simulink model "Corrado_simscape"  (R2023b)
settings: Solver=ode15s  StartTime=0.0  StopTime=15  RelTol=1e-2  AbsTol=1e-2  EnableMultiTasking=on
libraries: ee_lib x18, fl_lib x18, sm_lib x17, nesl_utility x7, simulink_extras x6
(part 2 of 2)

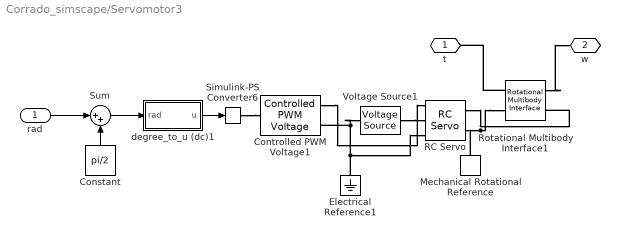
== system Corrado_simscape/Servomotor3 ==
  rad : Inport
  Constant : Constant  Value=pi/2
  Controlled PWM Voltage1 : ee_lib/Integrated Circuits/Controlled PWM Voltage  F=50 Hz  TD=0 s  pulse_width_offset=0 s  pulse_min=0 us  pwm_or_av=ee.enum.pwm_or_av.pwm  event_type=1  sample_time=5e-6 s  Vmin=0 V  Vmax=5 V  Vm=5 V  u_min=0  u_max=1
      settings: InternalSimscapePortConfiguration="{\"Bottom\":[],\"Left\":[{\"id\":\"u\",\"label\":\"u\",\"type\":\"input\"}],\"Right\":[{\"id\":\"p2\",\"label\":\"PWM\",\"type\":\"foundation.electrical.electrical\"},{\"id\":\"n2\",\"label\":\"REF\",\"type\":\"foundation.electrical.electrical\"}],\"Top\":[]}"
  Electrical Reference1 : fl_lib/Electrical/Electrical Elements/Electrical Reference
  Mechanical Rotational Reference : fl_lib/Mechanical/Rotational Elements/Mechanical Rotational Reference
  RC Servo : ee_lib/Electromechanical/Brushed Motors/RC Servo  stall_torque=15 cm*kg  time_60=0.13 s  nominal_voltage=6 V  rotational_range=[0, 180] deg  pulse_width_range=[600, 2400] us  threshold=3 V  R_s=18 kOhm  resolution=0.1 deg  angle_meas_error=0 deg  backdrive_torque=0.5 cm*kg  ratio=320  inertia=0.01 cm^2*g  endstop_angles=[-5, 185] deg  endstop_stiffness=1e6 N*m/rad  endstop_damping=0.01 N*m*s/rad  enable_faults=ee.enum.enable.no  fault_action=simscape.enum.assert.action.none  fault_type=ee.enum.electromech.rcservo.faultType.failOff  fault_trigger=ee.enum.faults.faultTrigger.temporal  t_fault=1 s  max_permissible_current=1 A  t_fail_on_current=1 s  angle_specify=off  angle_priority=High  angle=90 deg  angle_nominal_specify=off  angle_nominal_unit=deg  angle_nominal_value=1  w_specify=off  w_priority=High  w=0 deg/s  w_nominal_specify=off  w_nominal_unit=deg/s  w_nominal_value=1  torque_specify=off  torque_priority=None  torque=0 N*m  torque_nominal_specify=off  torque_nominal_unit=N*m  torque_nominal_value=1  pulse_width_specify=off  pulse_width_priority=Low  pulse_width=1.5 ms  i_specify=off  i_priority=None  i=0 A  i_nominal_specify=off  i_nominal_unit=A  i_nominal_value=1  i_s_specify=off  i_s_priority=None  i_s=0 A  i_s_nominal_specify=off  i_s_nominal_unit=A  i_s_nominal_value=1  motor_torque_specify=off  motor_torque_priority=None  motor_torque=0 N*m  motor_torque_nominal_specify=off  motor_torque_nominal_unit=N*m  motor_torque_nominal_value=1  power_dissipated_specify=off  power_dissipated_priority=None  power_dissipated=0 W  power_dissipated_nominal_specify=off  power_dissipated_nominal_unit=W  power_dissipated_nominal_value=1  angle_demand_specify=off  angle_demand_priority=None  angle_demand=90 deg  angle_demand_nominal_specify=off  angle_demand_nominal_unit=deg  angle_demand_nominal_value=1  faulted_specify=off  faulted_priority=None  faulted=0
      settings: InternalSimscapePortConfiguration="{\"Bottom\":[],\"Left\":[{\"id\":\"s\",\"label\":\"s\",\"type\":\"foundation.electrical.electrical\"},{\"id\":\"p\",\"label\":\"+\",\"type\":\"foundation.electrical.electrical\"},{\"id\":\"n\",\"label\":\"-\",\"type\":\"foundation.electrical.electrical\"}],\"Right\":[{\"id\":\"R\",\"label\":\"R\",\"type\":\"foundation.mechanical.rotational.rotational\"},{\"id\":\"C\",\"label\":\"C\",\"type\":\"foundation.mechanical.rotational.rotational\"}],\"Top\":[]}"
  Rotational Multibody Interface1 : fl_lib/Mechanical/Multibody Interfaces/Rotational Multibody Interface
  Simulink-PS Converter6 : nesl_utility/Simulink-PS Converter  PhysicalDomain=network_engine_domain  SubClassName=ps_input  LeftPortType=input  RightPortType=output  PseudoPeriodic=off  Frequencies=[]  NoiseDistribution=none  NoiseParameters=[]  Unit=1  AffineConversion=off  FilteringAndDerivatives=provide  SimscapeFilterOrder=1  InputFilterTimeConstant=0.001  UdotUserProvided=0
  Sum : Sum  Inputs=|++
  Voltage Source1 : ee_lib/Sources/Voltage Source  dc_voltage=6 V  ac_voltage=0 V  ac_shift=0 rad  ac_frequency=60 Hz  noise_mode=ee.enum.sources.noise.Disabled  PSD=0 V^2/Hz  sample_time=1e-3 s  repeatability=ee.enum.sources.repeatability.NotRepeatable  user_seed=0  auto_seed=4110765503  i_specify=off  i_priority=None  i=0 A  i_nominal_specify=off  i_nominal_unit=A  i_nominal_value=1  v_specify=off  v_priority=None  v=0 V  v_nominal_specify=off  v_nominal_unit=V  v_nominal_value=1
  degree_to_u (dc)1 : Subsystem
  t : PMIOPort  Side=Left
  w : PMIOPort  Port=2  Side=Right
  wires:
  degree_to_u (dc)1/1(u) -> Simulink-PS Converter6/1
  Constant/1 -> Sum/2
  rad/1 -> Sum/1
  Sum/1 -> degree_to_u (dc)1/1(rad)
  connections:
  Voltage Source1/RConn1 -- Controlled PWM Voltage1/RConn2 -- Electrical Reference1/LConn1 -- RC Servo/LConn3
  Simulink-PS Converter6/RConn1 -- Controlled PWM Voltage1/LConn1
  Controlled PWM Voltage1/RConn1 -- RC Servo/LConn1
  Voltage Source1/LConn1 -- RC Servo/LConn2
  Rotational Multibody Interface1/LConn1 -- t/RConn1
  Rotational Multibody Interface1/LConn2 -- RC Servo/RConn2 -- Mechanical Rotational Reference/LConn1
  RC Servo/RConn1 -- Rotational Multibody Interface1/RConn2
  Rotational Multibody Interface1/RConn1 -- w/RConn1

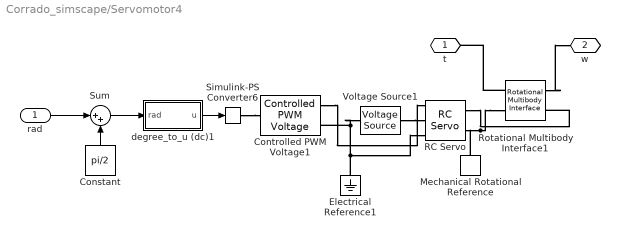
== system Corrado_simscape/Servomotor4 ==
  rad : Inport
  Constant : Constant  Value=pi/2
  Controlled PWM Voltage1 : ee_lib/Integrated Circuits/Controlled PWM Voltage  F=50 Hz  TD=0 s  pulse_width_offset=0 s  pulse_min=0 us  pwm_or_av=ee.enum.pwm_or_av.pwm  event_type=1  sample_time=5e-6 s  Vmin=0 V  Vmax=5 V  Vm=5 V  u_min=0  u_max=1
      settings: InternalSimscapePortConfiguration="{\"Bottom\":[],\"Left\":[{\"id\":\"u\",\"label\":\"u\",\"type\":\"input\"}],\"Right\":[{\"id\":\"p2\",\"label\":\"PWM\",\"type\":\"foundation.electrical.electrical\"},{\"id\":\"n2\",\"label\":\"REF\",\"type\":\"foundation.electrical.electrical\"}],\"Top\":[]}"
  Electrical Reference1 : fl_lib/Electrical/Electrical Elements/Electrical Reference
  Mechanical Rotational Reference : fl_lib/Mechanical/Rotational Elements/Mechanical Rotational Reference
  RC Servo : ee_lib/Electromechanical/Brushed Motors/RC Servo  stall_torque=15 cm*kg  time_60=0.13 s  nominal_voltage=6 V  rotational_range=[0, 180] deg  pulse_width_range=[600, 2400] us  threshold=3 V  R_s=18 kOhm  resolution=0.1 deg  angle_meas_error=0 deg  backdrive_torque=0.5 cm*kg  ratio=320  inertia=0.01 cm^2*g  endstop_angles=[-5, 185] deg  endstop_stiffness=1e6 N*m/rad  endstop_damping=0.01 N*m*s/rad  enable_faults=ee.enum.enable.no  fault_action=simscape.enum.assert.action.none  fault_type=ee.enum.electromech.rcservo.faultType.failOff  fault_trigger=ee.enum.faults.faultTrigger.temporal  t_fault=1 s  max_permissible_current=1 A  t_fail_on_current=1 s  angle_specify=off  angle_priority=High  angle=90 deg  angle_nominal_specify=off  angle_nominal_unit=deg  angle_nominal_value=1  w_specify=off  w_priority=High  w=0 deg/s  w_nominal_specify=off  w_nominal_unit=deg/s  w_nominal_value=1  torque_specify=off  torque_priority=None  torque=0 N*m  torque_nominal_specify=off  torque_nominal_unit=N*m  torque_nominal_value=1  pulse_width_specify=off  pulse_width_priority=Low  pulse_width=1.5 ms  i_specify=off  i_priority=None  i=0 A  i_nominal_specify=off  i_nominal_unit=A  i_nominal_value=1  i_s_specify=off  i_s_priority=None  i_s=0 A  i_s_nominal_specify=off  i_s_nominal_unit=A  i_s_nominal_value=1  motor_torque_specify=off  motor_torque_priority=None  motor_torque=0 N*m  motor_torque_nominal_specify=off  motor_torque_nominal_unit=N*m  motor_torque_nominal_value=1  power_dissipated_specify=off  power_dissipated_priority=None  power_dissipated=0 W  power_dissipated_nominal_specify=off  power_dissipated_nominal_unit=W  power_dissipated_nominal_value=1  angle_demand_specify=off  angle_demand_priority=None  angle_demand=90 deg  angle_demand_nominal_specify=off  angle_demand_nominal_unit=deg  angle_demand_nominal_value=1  faulted_specify=off  faulted_priority=None  faulted=0
      settings: InternalSimscapePortConfiguration="{\"Bottom\":[],\"Left\":[{\"id\":\"s\",\"label\":\"s\",\"type\":\"foundation.electrical.electrical\"},{\"id\":\"p\",\"label\":\"+\",\"type\":\"foundation.electrical.electrical\"},{\"id\":\"n\",\"label\":\"-\",\"type\":\"foundation.electrical.electrical\"}],\"Right\":[{\"id\":\"R\",\"label\":\"R\",\"type\":\"foundation.mechanical.rotational.rotational\"},{\"id\":\"C\",\"label\":\"C\",\"type\":\"foundation.mechanical.rotational.rotational\"}],\"Top\":[]}"
  Rotational Multibody Interface1 : fl_lib/Mechanical/Multibody Interfaces/Rotational Multibody Interface
  Simulink-PS Converter6 : nesl_utility/Simulink-PS Converter  PhysicalDomain=network_engine_domain  SubClassName=ps_input  LeftPortType=input  RightPortType=output  PseudoPeriodic=off  Frequencies=[]  NoiseDistribution=none  NoiseParameters=[]  Unit=1  AffineConversion=off  FilteringAndDerivatives=provide  SimscapeFilterOrder=1  InputFilterTimeConstant=0.001  UdotUserProvided=0
  Sum : Sum  Inputs=|++
  Voltage Source1 : ee_lib/Sources/Voltage Source  dc_voltage=6 V  ac_voltage=0 V  ac_shift=0 rad  ac_frequency=60 Hz  noise_mode=ee.enum.sources.noise.Disabled  PSD=0 V^2/Hz  sample_time=1e-3 s  repeatability=ee.enum.sources.repeatability.NotRepeatable  user_seed=0  auto_seed=3555390813  i_specify=off  i_priority=None  i=0 A  i_nominal_specify=off  i_nominal_unit=A  i_nominal_value=1  v_specify=off  v_priority=None  v=0 V  v_nominal_specify=off  v_nominal_unit=V  v_nominal_value=1
  degree_to_u (dc)1 : Subsystem
  t : PMIOPort  Side=Left
  w : PMIOPort  Port=2  Side=Right
  wires:
  degree_to_u (dc)1/1(u) -> Simulink-PS Converter6/1
  Constant/1 -> Sum/2
  rad/1 -> Sum/1
  Sum/1 -> degree_to_u (dc)1/1(rad)
  connections:
  Voltage Source1/RConn1 -- Controlled PWM Voltage1/RConn2 -- Electrical Reference1/LConn1 -- RC Servo/LConn3
  Simulink-PS Converter6/RConn1 -- Controlled PWM Voltage1/LConn1
  Controlled PWM Voltage1/RConn1 -- RC Servo/LConn1
  Voltage Source1/LConn1 -- RC Servo/LConn2
  Rotational Multibody Interface1/LConn1 -- t/RConn1
  Rotational Multibody Interface1/LConn2 -- RC Servo/RConn2 -- Mechanical Rotational Reference/LConn1
  RC Servo/RConn1 -- Rotational Multibody Interface1/RConn2
  Rotational Multibody Interface1/RConn1 -- w/RConn1

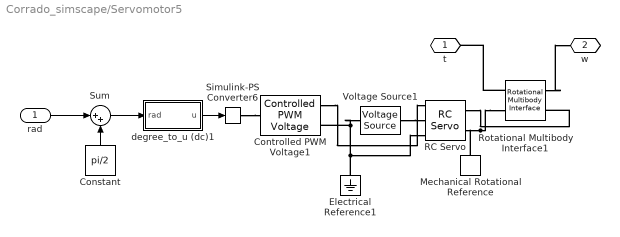
== system Corrado_simscape/Servomotor5 ==
  rad : Inport
  Constant : Constant  Value=pi/2
  Controlled PWM Voltage1 : ee_lib/Integrated Circuits/Controlled PWM Voltage  F=50 Hz  TD=0 s  pulse_width_offset=0 s  pulse_min=0 us  pwm_or_av=ee.enum.pwm_or_av.pwm  event_type=1  sample_time=5e-6 s  Vmin=0 V  Vmax=5 V  Vm=5 V  u_min=0  u_max=1
      settings: InternalSimscapePortConfiguration="{\"Bottom\":[],\"Left\":[{\"id\":\"u\",\"label\":\"u\",\"type\":\"input\"}],\"Right\":[{\"id\":\"p2\",\"label\":\"PWM\",\"type\":\"foundation.electrical.electrical\"},{\"id\":\"n2\",\"label\":\"REF\",\"type\":\"foundation.electrical.electrical\"}],\"Top\":[]}"
  Electrical Reference1 : fl_lib/Electrical/Electrical Elements/Electrical Reference
  Mechanical Rotational Reference : fl_lib/Mechanical/Rotational Elements/Mechanical Rotational Reference
  RC Servo : ee_lib/Electromechanical/Brushed Motors/RC Servo  stall_torque=15 cm*kg  time_60=0.13 s  nominal_voltage=6 V  rotational_range=[0, 180] deg  pulse_width_range=[600, 2400] us  threshold=3 V  R_s=18 kOhm  resolution=0.1 deg  angle_meas_error=0 deg  backdrive_torque=0.5 cm*kg  ratio=320  inertia=0.01 cm^2*g  endstop_angles=[-5, 185] deg  endstop_stiffness=1e6 N*m/rad  endstop_damping=0.01 N*m*s/rad  enable_faults=ee.enum.enable.no  fault_action=simscape.enum.assert.action.none  fault_type=ee.enum.electromech.rcservo.faultType.failOff  fault_trigger=ee.enum.faults.faultTrigger.temporal  t_fault=1 s  max_permissible_current=1 A  t_fail_on_current=1 s  angle_specify=off  angle_priority=High  angle=90 deg  angle_nominal_specify=off  angle_nominal_unit=deg  angle_nominal_value=1  w_specify=off  w_priority=High  w=0 deg/s  w_nominal_specify=off  w_nominal_unit=deg/s  w_nominal_value=1  torque_specify=off  torque_priority=None  torque=0 N*m  torque_nominal_specify=off  torque_nominal_unit=N*m  torque_nominal_value=1  pulse_width_specify=off  pulse_width_priority=Low  pulse_width=1.5 ms  i_specify=off  i_priority=None  i=0 A  i_nominal_specify=off  i_nominal_unit=A  i_nominal_value=1  i_s_specify=off  i_s_priority=None  i_s=0 A  i_s_nominal_specify=off  i_s_nominal_unit=A  i_s_nominal_value=1  motor_torque_specify=off  motor_torque_priority=None  motor_torque=0 N*m  motor_torque_nominal_specify=off  motor_torque_nominal_unit=N*m  motor_torque_nominal_value=1  power_dissipated_specify=off  power_dissipated_priority=None  power_dissipated=0 W  power_dissipated_nominal_specify=off  power_dissipated_nominal_unit=W  power_dissipated_nominal_value=1  angle_demand_specify=off  angle_demand_priority=None  angle_demand=90 deg  angle_demand_nominal_specify=off  angle_demand_nominal_unit=deg  angle_demand_nominal_value=1  faulted_specify=off  faulted_priority=None  faulted=0
      settings: InternalSimscapePortConfiguration="{\"Bottom\":[],\"Left\":[{\"id\":\"s\",\"label\":\"s\",\"type\":\"foundation.electrical.electrical\"},{\"id\":\"p\",\"label\":\"+\",\"type\":\"foundation.electrical.electrical\"},{\"id\":\"n\",\"label\":\"-\",\"type\":\"foundation.electrical.electrical\"}],\"Right\":[{\"id\":\"R\",\"label\":\"R\",\"type\":\"foundation.mechanical.rotational.rotational\"},{\"id\":\"C\",\"label\":\"C\",\"type\":\"foundation.mechanical.rotational.rotational\"}],\"Top\":[]}"
  Rotational Multibody Interface1 : fl_lib/Mechanical/Multibody Interfaces/Rotational Multibody Interface
  Simulink-PS Converter6 : nesl_utility/Simulink-PS Converter  PhysicalDomain=network_engine_domain  SubClassName=ps_input  LeftPortType=input  RightPortType=output  PseudoPeriodic=off  Frequencies=[]  NoiseDistribution=none  NoiseParameters=[]  Unit=1  AffineConversion=off  FilteringAndDerivatives=provide  SimscapeFilterOrder=1  InputFilterTimeConstant=0.001  UdotUserProvided=0
  Sum : Sum  Inputs=|++
  Voltage Source1 : ee_lib/Sources/Voltage Source  dc_voltage=6 V  ac_voltage=0 V  ac_shift=0 rad  ac_frequency=60 Hz  noise_mode=ee.enum.sources.noise.Disabled  PSD=0 V^2/Hz  sample_time=1e-3 s  repeatability=ee.enum.sources.repeatability.NotRepeatable  user_seed=0  auto_seed=442554284  i_specify=off  i_priority=None  i=0 A  i_nominal_specify=off  i_nominal_unit=A  i_nominal_value=1  v_specify=off  v_priority=None  v=0 V  v_nominal_specify=off  v_nominal_unit=V  v_nominal_value=1
  degree_to_u (dc)1 : Subsystem
  t : PMIOPort  Side=Left
  w : PMIOPort  Port=2  Side=Right
  wires:
  degree_to_u (dc)1/1(u) -> Simulink-PS Converter6/1
  Constant/1 -> Sum/2
  rad/1 -> Sum/1
  Sum/1 -> degree_to_u (dc)1/1(rad)
  connections:
  Voltage Source1/RConn1 -- Controlled PWM Voltage1/RConn2 -- Electrical Reference1/LConn1 -- RC Servo/LConn3
  Simulink-PS Converter6/RConn1 -- Controlled PWM Voltage1/LConn1
  Controlled PWM Voltage1/RConn1 -- RC Servo/LConn1
  Voltage Source1/LConn1 -- RC Servo/LConn2
  Rotational Multibody Interface1/LConn1 -- t/RConn1
  Rotational Multibody Interface1/LConn2 -- RC Servo/RConn2 -- Mechanical Rotational Reference/LConn1
  RC Servo/RConn1 -- Rotational Multibody Interface1/RConn2
  Rotational Multibody Interface1/RConn1 -- w/RConn1

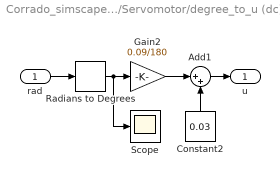
== system Corrado_simscape/Servomotor/degree_to_u (dc)1 ==
  rad : Inport
  Add1 : Sum  Inputs=|++
  Constant2 : Constant  Value=0.03
  Gain2 : Gain  Gain=0.09/180
  Radians to Degrees : simulink_extras/Transformations/Radians to Degrees
  Scope : Scope
  u : Outport
  wires:
  rad/1 -> Radians to Degrees/1
  Constant2/1 -> Add1/2
  Gain2/1 -> Add1/1
  Add1/1 -> u/1
  Radians to Degrees/1 -> Scope/1, Gain2/1

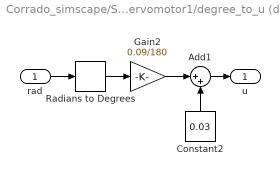
== system Corrado_simscape/Servomotor1/degree_to_u (dc)1 ==
  rad : Inport
  Add1 : Sum  Inputs=|++
  Constant2 : Constant  Value=0.03
  Gain2 : Gain  Gain=0.09/180
  Radians to Degrees : simulink_extras/Transformations/Radians to Degrees
  u : Outport
  wires:
  rad/1 -> Radians to Degrees/1
  Constant2/1 -> Add1/2
  Gain2/1 -> Add1/1
  Add1/1 -> u/1
  Radians to Degrees/1 -> Gain2/1

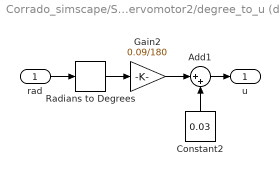
== system Corrado_simscape/Servomotor2/degree_to_u (dc)1 ==
  rad : Inport
  Add1 : Sum  Inputs=|++
  Constant2 : Constant  Value=0.03
  Gain2 : Gain  Gain=0.09/180
  Radians to Degrees : simulink_extras/Transformations/Radians to Degrees
  u : Outport
  wires:
  rad/1 -> Radians to Degrees/1
  Constant2/1 -> Add1/2
  Gain2/1 -> Add1/1
  Add1/1 -> u/1
  Radians to Degrees/1 -> Gain2/1

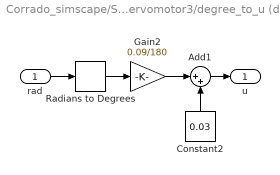
== system Corrado_simscape/Servomotor3/degree_to_u (dc)1 ==
  rad : Inport
  Add1 : Sum  Inputs=|++
  Constant2 : Constant  Value=0.03
  Gain2 : Gain  Gain=0.09/180
  Radians to Degrees : simulink_extras/Transformations/Radians to Degrees
  u : Outport
  wires:
  rad/1 -> Radians to Degrees/1
  Constant2/1 -> Add1/2
  Gain2/1 -> Add1/1
  Add1/1 -> u/1
  Radians to Degrees/1 -> Gain2/1

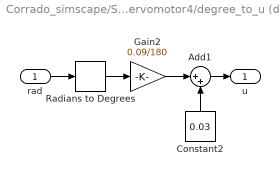
== system Corrado_simscape/Servomotor4/degree_to_u (dc)1 ==
  rad : Inport
  Add1 : Sum  Inputs=|++
  Constant2 : Constant  Value=0.03
  Gain2 : Gain  Gain=0.09/180
  Radians to Degrees : simulink_extras/Transformations/Radians to Degrees
  u : Outport
  wires:
  rad/1 -> Radians to Degrees/1
  Constant2/1 -> Add1/2
  Gain2/1 -> Add1/1
  Add1/1 -> u/1
  Radians to Degrees/1 -> Gain2/1

== system Corrado_simscape/Servomotor5/degree_to_u (dc)1 ==
  rad : Inport
  Add1 : Sum  Inputs=|++
  Constant2 : Constant  Value=0.03
  Gain2 : Gain  Gain=0.09/180
  Radians to Degrees : simulink_extras/Transformations/Radians to Degrees
  u : Outport
  wires:
  rad/1 -> Radians to Degrees/1
  Constant2/1 -> Add1/2
  Gain2/1 -> Add1/1
  Add1/1 -> u/1
  Radians to Degrees/1 -> Gain2/1
